simulink library "wt_blockset_beta"  (Simulink 5.0)
values from neighbouring files (symbols this model uses):
  a = -Le\Re    [matrix_coeff_trafo3limb_abc.m]
  a11 = K2*Rs/Ls    [matrix_coeff_scim_abc.m]    (also in matrix_coeff_spsm_dq.m = -Rs*Ksgm_frd/Ksgm_d; matrix_coeff_trafo_abc.m = K2*Rhv/Lhv; matrix_coeff_wrim_abc.m)
  a12 = K3*Rs/Ls    [matrix_coeff_scim_abc.m]    (also in matrix_coeff_spsm_dq.m = Lssq*Ksgm_frd/Ksgm_d; matrix_coeff_trafo_abc.m = K3*Rhv/Lhv; matrix_coeff_wrim_abc.m)
  a13 = 3*Msr*sqrt(3)*K4/4    [matrix_coeff_scim_abc.m]    (also in matrix_coeff_spsm_dq.m = Rf*Lsgm_rd*Lmd/Ksgm_d; matrix_coeff_trafo_abc.m = K4*Rhv; matrix_coeff_wrim_abc.m)
  a14 = K4*Rr    [matrix_coeff_scim_abc.m]    (also in matrix_coeff_spsm_dq.m = Rrd*Lsgm_f*Lmd/Ksgm_d; matrix_coeff_trafo_abc.m = K2/Lhv; matrix_coeff_wrim_abc.m)
  a15 = Msr*(K2-K3)/Ls    [matrix_coeff_scim_abc.m]    (also in matrix_coeff_spsm_dq.m = Lmq*Ksgm_frd/Ksgm_d; matrix_coeff_trafo_abc.m = K3/Lhv; matrix_coeff_wrim_abc.m)
  a16 = K2/Ls    [matrix_coeff_scim_abc.m]    (also in matrix_coeff_spsm_dq.m = Ksgm_frd/Ksgm_d; matrix_coeff_trafo_abc.m = K4; matrix_coeff_wrim_abc.m)
  a17 = K3/Ls    [matrix_coeff_scim_abc.m]    (also in matrix_coeff_spsm_dq.m = -Lsgm_rd*Lmd/Ksgm_d; matrix_coeff_wrim_abc.m)
  a21 = -Lssd*Lsrq/Ksgm_q    [matrix_coeff_spsm_dq.m]
  a22 = -Rs*Lsrq/Ksgm_q    [matrix_coeff_spsm_dq.m]
  a23 = -Lsrq*Lmd/Ksgm_q    [matrix_coeff_spsm_dq.m]
  a24 = -Lsrq*Lmd/Ksgm_q    [matrix_coeff_spsm_dq.m]
  a25 = Rrq*Lmq/Ksgm_q    [matrix_coeff_spsm_dq.m]
  a26 = Lsrq/Ksgm_q    [matrix_coeff_spsm_dq.m]
  a31 = K4*Rs    [matrix_coeff_scim_abc.m]    (also in matrix_coeff_spsm_dq.m = +Rs*Lsgm_rd*Lmd/Ksgm_d; matrix_coeff_trafo_abc.m = K4*Rlv; matrix_coeff_wrim_abc.m)
  a32 = Msr*(K2-K3)/Lr    [matrix_coeff_scim_abc.m]    (also in matrix_coeff_spsm_dq.m = -Lssq*Lsgm_rd*Lmd/Ksgm_d; matrix_coeff_trafo_abc.m = K2*Rlv/Llv; matrix_coeff_wrim_abc.m)
  a33 = K2*Rr/Lr    [matrix_coeff_scim_abc.m]    (also in matrix_coeff_spsm_dq.m = -Rf*Ksgm_srd/Ksgm_d; matrix_coeff_trafo_abc.m = K3*Rlv/Llv; matrix_coeff_wrim_abc.m)
  a34 = K3*Rr/Lr    [matrix_coeff_scim_abc.m]    (also in matrix_coeff_spsm_dq.m = Rrd*Lsgm_s*Lmd/Ksgm_d; matrix_coeff_trafo_abc.m = K4; matrix_coeff_wrim_abc.m)
  a35 = 3*Msr*sqrt(3)*K4/4    [matrix_coeff_scim_abc.m]    (also in matrix_coeff_spsm_dq.m = -Lsgm_rd*Lmd*Lmq/Ksgm_d; matrix_coeff_trafo_abc.m = K2/Llv; matrix_coeff_wrim_abc.m)
  a36 = K4    [matrix_coeff_scim_abc.m]    (also in matrix_coeff_spsm_dq.m = -Lsgm_rd*Lmd/Ksgm_d; matrix_coeff_trafo_abc.m = K3/Llv; matrix_coeff_wrim_abc.m)
  a37 = Ksgm_srd/Ksgm_d    [matrix_coeff_spsm_dq.m]    (also in matrix_coeff_wrim_abc.m = K2/Lr)
  a41 = Rs*Lsgm_f*Lmd/Ksgm_d    [matrix_coeff_spsm_dq.m]
  a42 = -Lsgm_f*Lssq*Lmd/Ksgm_d    [matrix_coeff_spsm_dq.m]
  a43 = Rf*Lsgm_s*Lmd/Ksgm_d    [matrix_coeff_spsm_dq.m]
  a44 = -Rrd*Ksgm_sf/Ksgm_d    [matrix_coeff_spsm_dq.m]
  a45 = -Lsgm_f*Lmd*Lmq/Ksgm_d    [matrix_coeff_spsm_dq.m]
  a46 = -Lsgm_f*Lmd/Ksgm_d    [matrix_coeff_spsm_dq.m]
  a47 = -Lsgm_s*Lmd/Ksgm_d    [matrix_coeff_spsm_dq.m]
  a51 = Lssd*Lmq/Ksgm_q    [matrix_coeff_spsm_dq.m]
  a52 = Rs*Lmq/Ksgm_q    [matrix_coeff_spsm_dq.m]
  a53 = Lmd*Lmq/Ksgm_q    [matrix_coeff_spsm_dq.m]
  a54 = Lmd*Lmq/Ksgm_q    [matrix_coeff_spsm_dq.m]
  a55 = -Rrq*Lssq/Ksgm_q    [matrix_coeff_spsm_dq.m]
  a56 = -Lmq/Ksgm_q    [matrix_coeff_spsm_dq.m]
  alpha_T = Ubase_hv/Ubase_lv    [matrix_coeff_trafo3limb_abc.m]
  b = inv(Le)    [matrix_coeff_trafo3limb_abc.m]
  Ctorque = cq(2:5:102,2:5:182)    [cq_table.m]
  Lmd = mag_ind(1)    [matrix_coeff_spsm_dq.m]
  Lmq = mag_ind(2)    [matrix_coeff_spsm_dq.m]
  Lss = Lsgms+Lm    [init_dbe_dq_scim.m]
  omg_base = 2*pi*rated_fp(1)    [init_dbe_dq_scim.m]    (also in init_dbe_rms_scim.m)
  p = rated_fp(2)    [init_dbe_dq_scim.m]    (also in init_dbe_rms_scim.m)
  Rs = stator(1)    [init_dbe_dq_scim.m]    (also in init_dbe_rms_scim.m; matrix_coeff_scim_abc.m; matrix_coeff_spsm_dq.m = stator_winding(1); matrix_coeff_wrim_abc.m)
  Xs = omg_base*Lss    [init_dbe_dq_scim.m]    (also in init_dbe_rms_scim.m = Xsgm_s+Xm)
undefined symbols (not defined in the file or in its folder): get, j, Kmode, ModeOp, Type, u0
libraries: simulink_extras x12, simulink x4, dspinverses x1, dspmtrx3 x1, dspsigattribs x1, dspspect3 x1
(part 1 of 4)
settings Model: Creator=Florin iov  LastModifiedBy=fi  ModifiedComment=fi -- Tue Jun 01 12:17:17 2004 -- Version beta 1

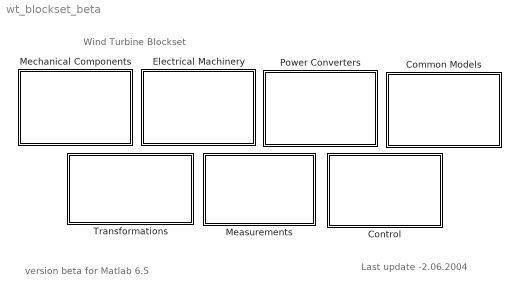
== system wt_blockset_beta ==
  note: Wind Turbine Blockset
  note: Last update -2.06.2004
  note: version beta for Matlab 6.5
  Common Models : Subsystem
      mask Display: disp('Common\nModels')
  Control : Subsystem
      mask Display: disp('Control')
  Electrical Machinery : Subsystem
      mask Display: disp('Electrical\nMachinery')
  Measurements : Subsystem
      mask Display: disp('Measurements')
  Mechanical Components : Subsystem
      mask Display: disp('Mechanical\nComponents')
  Power Converters : Subsystem
      mask Display: disp('Power\nConverters')
  Transformations : Subsystem
      mask Display: disp('Transformations')

== system wt_blockset_beta/Common Models ==
  note: Sources
  note: Cables & Distribution Lines
  note: others
  note: Transformers
  3-phase 3 limb  C S-Function : Subsystem  mask(ABC/abc Dynamic Model of 3-phase 3 limb transformer){power=[2e6 3000], voltage=[30000 690/sqrt(3)], frequency=50, hv_winding=[4.5 51], lv_winding=[3 51], core_ratio=0.33}
      mask prompts: power "Rated power, No-load losses [Sr (VA), Po (W)]"; voltage "Rated phase voltages [U1r (V), U2r (V)]]"; frequency "Rated frequency [Hz]"; hv_winding "High-voltage windings [Rhv  X_hv] [ohms]"; lv_winding "Low-voltage windings [Rlv X_lv] [ohms]"; core_ratio "Core ratio (l/L)"
      mask help:
      | Implements a dynamic model of a 3-phase 2-windings transformer in natural frame (ABC/abc). Core geometry is taken into account.
      | Connection Type Dyn1.
      mask init:
      | matrix_coeff_trafo3limb_abc
      | init_cond = [0 0 0 0 0 0];
      mask Display: disp('3phase 3 limb\n Transformer')
  3-phase 3 limb  Transformer : Subsystem  mask(ABC/abc Dynamic Model of 3-phase 3 limb transformer){power=[2e6 3000], voltage=[30000 690/sqrt(3)], frequency=50, hv_winding=[4.5 51], lv_winding=[3 51], core_ratio=0.33}
      mask prompts: power "Rated power, No-load losses [Sr (VA), Po (W)]"; voltage "Rated phase voltages [U1r (V), U2r (V)]]"; frequency "Rated frequency [Hz]"; hv_winding "High-voltage windings [Rhv  X_hv] [ohms]"; lv_winding "Low-voltage windings [Rlv X_lv] [ohms]"; core_ratio "Core ratio (l/L)"
      mask help:
      | Implements a dynamic model of a 3-phase 2-windings transformer in natural frame (ABC/abc). Core geometry is taken into account.
      | Connection Type Dyn1.
      mask init:
      | matrix_coeff_trafo3limb_abc
      mask Display: disp('3phase 3 limb\n Transformer')
  3-phase line : Subsystem  mask(3-phase distribution line){d=3.3, R=0.115, L=0.19/314, C=0.52e-6}
      mask prompts: d "Line length [km]"; R "Line resistance [ohms/km]"; L "Line inductance [H/km]"; C "Line capacitance [F/km]"
      mask init:
      | Zc=sqrt(L/C);
      | tdelay=d*sqrt(L*C);
      | atten=exp(-(R/2)*d*sqrt(C/L));
      | buffer_size=20000;
  3-phase source : Subsystem  mask(3 - Phase Voltage Source){Uf=220, fs=50}
      mask prompts: Uf "Phase voltage [V]"; fs "Fundamental frequency [Hz]"
  Capacitor Bank RC : Subsystem  mask(Capacitor Bank RC){R=1, CmF=21.737}
      mask prompts: R "Series rezistor [ohms]"; CmF "Branch Capacitor [mF]"
      mask init:
      | C=CmF*1e-3;
      mask Display: disp('Capacitor\nBank')
  Capacitor Bank RLC : Subsystem  mask(Capacitor Bank RLC){R=0.0001, X=0.00034, CmF=0.0005}
      mask prompts: R "Series rezistor [ohms]"; X "Reactor [ohms]"; CmF "Capacitance [mF]"
      mask init:
      | L=X/(2*pi*50);
      | C=CmF*1e-3;
      mask Display: disp('Capacitor\nBank')
  Circuit breaker : Subsystem  mask{to=1/50, Ro=100, tc=1/50, Rc=100}
      mask prompts: to "Opening time"; Ro "Opening resistance"; tc "Closing time"; Rc "Closing resistance"
  DC-link circuit : Subsystem  mask(DC-link circuit){R=0.001, CuF=21.737}
      mask prompts: R "Series rezistor [ohms]"; CuF "Capacitor [uF]"
      mask init:
      | C=CuF*1e-6;
      mask Display: disp('DC\nLink')
  GRID 1 : Subsystem  mask(3 - Phase Voltage Source){Uf=31500, R=0, X=1.5, fs=50}
      mask prompts: Uf "Phase voltage [V]"; R "Resistance"; X "Reactance"; fs "Fundamental frequency [Hz]"
  GRID 2 : Subsystem  mask(3 - Phase Voltage Source){Uf=31500, R=0.01, X=5, fs=50}
      mask prompts: Uf "Phase voltage [V]"; R "Resistance"; X "Reactance"; fs "Fundamental frequency [Hz]"
  Harmonic Voltage Source : Subsystem  mask(Harmonic Voltage Source){phase_o=178.2, h3=on, h5=on, h7=on, h9=on, h11=on, h13=on}
      mask prompts: phase_o "Initial phase [deg]"; h3 "Insertion of 3rd harmonic"; h5 "Insertion of 5th harmonic"; h7 "Insertion of 7th harmonic"; h9 "Insertion of 9th harmonic"; h11 "Insertion of 11th harmonic"; h13 "Insertion of 13th harmonic"
      mask help: Implements a harmonic voltage source according with Standard EN61000-2-2.
      mask init:
      | gama_0=phase_o*pi/180;
  Voltage source complex : Subsystem  mask(3 - Phase Voltage Source){Uf=960}
      mask prompts: Uf "Phase voltage [V]"

== system wt_blockset_beta/Control ==
  note: Control Blocks
  PI anti wind-up : Subsystem  mask{K=0.09, Ti=0.016, ka=10, maxim=1000, init_cond=2}
      mask prompts: K "Proportional Constant"; Ti "Integrate constant"; maxim "Limits"; init_cond "initial"

== system wt_blockset_beta/Electrical Machinery ==
  note: Electrical Machinery Library
  Simulink Blocks  based Models : Subsystem
      mask Display: disp('Simulink Blocks\n based Models')

== system wt_blockset_beta/Measurements ==
  note: Measurements
  Moving Average Filter : Subsystem  mask(Moving Average Filter){Tav=60, init=10}
      mask prompts: Tav "Averaging time interval [sec]"; init "Initial condition"
      mask help: Implements a Moving average filter in time domain
      mask Display: disp('Moving\nAverage')
  P & Q three phase : Subsystem  mask(Active & Reactive Power ){f=50}
      mask prompts: f "Fundamental frequency (Hz):"
      mask Display: disp('P&Q\n 3-phase')
  Phase Locked Loop : Subsystem  mask(Phase Locked Loop){fs=50, Kp=180.03, Ti=0.00786}
      mask prompts: fs "Fundamental frequency (Hz):"; Kp "Proportional coefficient"; Ti "Integration time constant [sec]"
      mask help: Implements a Phase Locked Loop for grid angle detection
      mask Display: disp('PLL')
  power spectra : Subsystem  mask(power spectra){t_sample=0.05}
      mask prompts: t_sample "Sample period"

== system wt_blockset_beta/Mechanical Components ==
  note: Wind Models
  note: Drive Train Models
  note: Rotor Models
  "One-mass model " : Subsystem  mask(Simple Gearbox){Op_Mode=Generator, Jem=90, Jwt=9e6, K=83, init_speed=1.87355}
      mask prompts: Op_Mode "Operation Mode"; Jem "Electric machinery - Moment of inertia [kg m2]"; Jwt "Wind turbine rotor - Moment of inertia [kg*m2]"; K "Gearbox ratio"; init_speed "Initial condition [omg_wt (rad/sec)]"
      mask init:
      | if Op_Mode==1, ModeOp=-1;else ModeOp=1;end
      | J=Jem*K^2+Jwt;
      mask StyleString: popup(Motor|Generator),edit,edit,edit,edit
      mask Display: disp('Drive Train')
  Two-mass model : Subsystem  mask(Gearbox with torsional torque){Jem=90, Jwt=9e6, Kshaft=12e7, Dshaft=3.5e5, Kgear=83, init=[156.5 1.87355]}
      mask prompts: Jem "Electric machine - Moment of inertia:  Jem [ kg*m2]"; Jwt "Wind turbine rotor - Moment of inertia:  Jwt [kg*m2]"; Kshaft "Shaft stiffness:  Kshaft [ Nm/rad]"; Dshaft "Damping coeficient of shaft:  Dshaft [Nm sec/rad]"; Kgear "Gearbox ratio"; init "Initial conditions [omg_em (rad/sec), omg_wt (rad/sec) ]"
      mask help: Implements a gearbox with torsional torque.
      mask Display: disp('Drive Train')
  Two-mass model 'C' S-Function : Subsystem  mask(Gear box with torsional torques){Jem=90, Jwt=9e6, Kshaft=12e7, Dshaft=3.5e5, Kgear=83, init_cond=[156.5 0 1.87355 0]}
      mask prompts: Jem "Electric machine - Moment of inertia:  Jem [ kg*m2]"; Jwt "Wind turbine rotor - Moment of inertia:  Jwt [kg*m2]"; Kshaft "Shaft stiffness:  Kshaft [ Nm/rad]"; Dshaft "Damping coeficient of shaft:  Dshaft [Nm sec/rad]"; Kgear "Gearbox ratio"; init_cond "Initial conditions [omg_em(rad/s) th_em(rad) omg_wtr(rad/s) th_wtr(rad)]"
      mask help:
      | Implemets the dynamic model of a gearbox with torsional torques.
      | Equations are written at the low speed shaft (wind turbine side).
      mask Display: disp('Drive Train')
  Wind Model SB-1 : Subsystem  TreatAsAtomicUnit=on  mask(Wind Model using Simulink Band-limited white noise generator){D_rotor=72, v_mean=10, roughness=600, turb_int=12, T_sample=0.05}
      mask prompts: D_rotor "Rotor diameter [m]"; v_mean "Average wind speed [m/sec]"; roughness "Length scale [m]"; turb_int "Turbulence intensity [%]"; T_sample "Sample time [sec]"
      mask help:
      | Implements a rotor wind model developped by RISOE National Laboratory based on Kaimal spectra. The model takes into account the rotational turbulences and the tower shadow.
      | This model uses the built-in band-limited white noise generator from Simulink
      mask init:
      | r = D_rotor/2;
      | sigma = v_mean*turb_int/100;
      | var = sigma^2;
      | c = roughness/(2*pi*v_mean);
      | d = r/v_mean;
      | trans=sigma*sqrt(roughness/v_mean);
      mask Display: disp('Wind\nModel\n(SB-1)')
  Wind Model SB-2 : Subsystem  TreatAsAtomicUnit=on  mask(Wind Model using Simulink Band-limited white noise generator){D_rotor=72, L=600, turb_int=12, T_sample=0.05}
      mask prompts: D_rotor "Rotor diameter [m]"; L "Length scale [m]"; turb_int "Turbulence intensity [%]"; T_sample "Sample time [sec]"
      mask help:
      | Implements a rotor wind model developped by RISOE National Laboratory based on Kaimal spectra. The model takes into account the rotational turbulences and the tower shadow.
      | This model uses the built-in band-limited white noise generator from Simulink
      mask init:
      | r = D_rotor/2;
      mask Display: disp('Wind\nModel\n(SB-2)')
  Wind Turbine Rotor : Subsystem  mask(Aerodynamic model for wind turbine){R=40, ro_air=1.25, cut_in=3, cut_out=25, Tact=0}
      mask prompts: R "Blade radius [m]"; ro_air "Air density [kg m3]"; cut_in "Cut in speed [m/sec]"; cut_out "Cut out speed [m/sec]"; Tact "Time constant for pitch actuator [sec]"
      mask init:
      | cq_table
      mask Display: plot(20,0,120,200,[45,35,35,45,75,75,45],[85,92,108,115,115,85,85],[55,50,70,65],[115,180,190,115],[55,50,70,65],[85,10,20,85],[75,85],[102,102],[75,85],[98,98],[105,85,85,105],[80,85,115,120])

== system wt_blockset_beta/Power Converters ==
  note: Power Converters Models
  note: Modulation Strategies
  3-phase Diode Bridge Rectifier : Subsystem
      mask Type: 3 phase Diode Bridge Rectifier
      mask Description: Implements a model for 3 phase Diode Bridge Rectifier.
      mask Display: disp('')
  Average PWM Strategy : Subsystem  mask(Average sinusoidal PWM Strategy with Simulink Blocks){third=on}
      mask prompts: third "Insertion of third harmonic"
      mask help: Implements an average model of a sinusoidal PWM strategy using Simulink Blocks.
      mask Display: disp('Average\nPWM')
  Average SVM Strategy : Subsystem
      mask Type: Average SVM Strategy with Simulink Blocks
      mask Description: Implements an average model of a SV-PWM strategy using Simulink Blocks.
      mask Display: disp('Average\nSVM')
  Switching PWM Strategy : Subsystem  mask(Switching sinusoidal PWM with Simulink Blocks){carrier=1000, dead_time=3.2e-6, min_pw=5e-6, dp=on, third=on}
      mask prompts: carrier "Carrier frequency [Hz]"; dead_time "Dead time [sec]"; min_pw "Minimum pulse width [sec]"; dp "Pulse dropping"; third "Insertion of third harmonic"
      mask help: Implements a switching model of a sinusoidal PWM strategy using Simulink Blocks.
      mask init:
      | mpw=0.5*min_pw;
      mask Display: disp('Switching\nPWM')
  Switching SVM Strategy : Subsystem  mask(Switching SVM Strategy with Simulink Blocks){fsw=4000, dead_time=3.2e-6, min_pw=5e-6, dp=off}
      mask prompts: fsw "Switching frequency"; dead_time "Dead time [sec]"; min_pw "Minimum pulse width [sec]"; dp "Pulse dropping"
      mask help: Implements a switching model of a SV-PWM strategy using Simulink Blocks.
      mask init:
      | Tsw=1/fsw;
      | mpw=0.5*min_pw;
      mask Display: disp('Switching\nSVM')
  Voltage Source Converter : Subsystem
      mask Type: Voltage Source Converter - star connected loads
      mask Description:
      | Implements a Voltage Source Converter (Rectifier or Inverter)
      | using switching functions.
      | - input S_ABC is          discret (0,1) => switching model.
      | - input S_ABC is continuous (0...1) =>   average model.
      mask Display: disp('VSC')

== system wt_blockset_beta/Transformations ==
  note: Transformations
  ABC->Mag&Phase : Subsystem
      mask Type: RMS&phase calculator
      mask Description: Calculate the RMS value and phase angle for a 3 phase input.
      mask Display: disp('')
  "DQ -> Complex" : Subsystem
      mask Type: DQ -> Complex
      mask Description: Transformation of dq variables into complex form
  "abc -> dq0" : Subsystem
      mask Description: Implements  ABC -> DQ  transformation
  "dq0 -> abc" : Subsystem
      mask Type: DQ -> ABC
      mask Description: Implements DQ -> ABC transformation
      mask Display: disp(' ')
  "phase -> line currents" : Subsystem
      mask Type: Transformation phase to line currents
      mask Description: Transformation of phase currents into line currents
      mask Display: disp('')
  phase->line voltages : Subsystem
      mask Type: Transformation phase to line voltages
      mask Description: Transformation of phase currents into line voltages
      mask Display: disp('')

== system wt_blockset_beta/Common Models/3-phase 3 limb  C S-Function ==
  v_UVW : Inport
  i_uvw : Inport  Port=2
  Mux : Mux  Inputs=2
  Ropen : Gain  Orientation=down  Gain=1000000  SaturateOnIntegerOverflow=on
  Ropen1 : Gain  Gain=-sqrt(3)  SaturateOnIntegerOverflow=on
  S-Function : S-Function  FunctionName=trafo3limb_abc  Parameters=a b init_cond
  Selector iABC : Selector  Elements=[1 2 3]  InputPortWidth=6
  Selector iabc : Selector  Elements=[4 5 6]  InputPortWidth=6
  Sum : Sum  Inputs=|+-  SaturateOnIntegerOverflow=on  InputSameDT=on
  phase->line2 : Subsystem
  turns ratio : Gain  Gain=-alpha_T  SaturateOnIntegerOverflow=on
  turns ratio1 : Gain  Gain=alpha_T  SaturateOnIntegerOverflow=on
  i_UVW : Outport
  v_uvw : Outport  Port=2
  wires:
  i_uvw/1 -> Sum/2
  turns ratio1/1 -> Sum/1
  Ropen1/1 -> v_uvw/1
  Ropen/1 -> turns ratio/1, Ropen1/1
  Sum/1 -> Ropen/1
  S-Function/1 -> Selector iabc/1, Selector iABC/1
  Mux/1 -> S-Function/1
  turns ratio/1 -> Mux/2
  v_UVW/1 -> Mux/1
  phase->line2/1(out) -> i_UVW/1
  Selector iABC/1 -> phase->line2/1(in)
  Selector iabc/1 -> turns ratio1/1

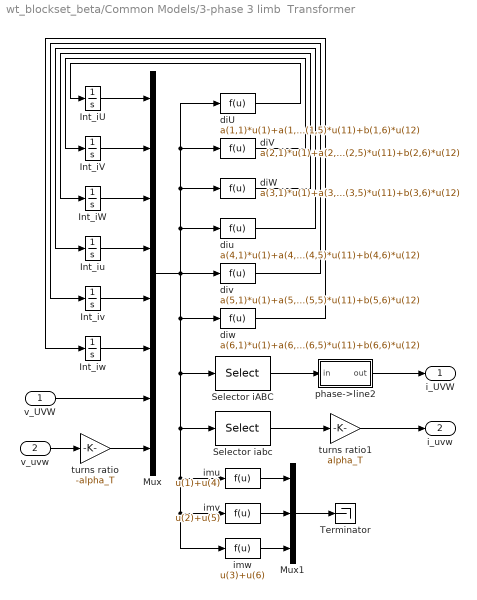
== system wt_blockset_beta/Common Models/3-phase 3 limb  Transformer ==
  v_UVW : Inport
  v_uvw : Inport  Port=2
  Int_iU : Integrator
  Int_iV : Integrator
  Int_iW : Integrator
  Int_iu : Integrator
  Int_iv : Integrator
  Int_iw : Integrator
  Mux : Mux  Inputs=[1 1 1 1 1 1 3 3]
  Mux1 : Mux  Inputs=3
  Selector iABC : Selector  Elements=[1 2 3]  InputPortWidth=12
  Selector iabc : Selector  Elements=[4 5 6]  InputPortWidth=12
  Terminator : Terminator
  diU : Fcn  Expr=a(1,1)*u(1)+a(1,2)*u(2)+a(1,3)*u(3)+a(1,4)*u(4)+a(1,5)*u(5)+a(1,6)*u(6)+b(1,1)*u(7)+b(1,2)*u(8)+b(1,3)*u(9)+b(1,4)*u(10)+b(1,5)*u(11)+b(1,6)*u(12)
  diV : Fcn  Expr=a(2,1)*u(1)+a(2,2)*u(2)+a(2,3)*u(3)+a(2,4)*u(4)+a(2,5)*u(5)+a(2,6)*u(6)+b(2,1)*u(7)+b(2,2)*u(8)+b(2,3)*u(9)+b(2,4)*u(10)+b(2,5)*u(11)+b(2,6)*u(12)
  diW : Fcn  Expr=a(3,1)*u(1)+a(3,2)*u(2)+a(3,3)*u(3)+a(3,4)*u(4)+a(3,5)*u(5)+a(3,6)*u(6)+b(3,1)*u(7)+b(3,2)*u(8)+b(3,3)*u(9)+b(3,4)*u(10)+b(3,5)*u(11)+b(3,6)*u(12)
  diu : Fcn  Expr=a(4,1)*u(1)+a(4,2)*u(2)+a(4,3)*u(3)+a(4,4)*u(4)+a(4,5)*u(5)+a(4,6)*u(6)+b(4,1)*u(7)+b(4,2)*u(8)+b(4,3)*u(9)+b(4,4)*u(10)+b(4,5)*u(11)+b(4,6)*u(12)
  div : Fcn  Expr=a(5,1)*u(1)+a(5,2)*u(2)+a(5,3)*u(3)+a(5,4)*u(4)+a(5,5)*u(5)+a(5,6)*u(6)+b(5,1)*u(7)+b(5,2)*u(8)+b(5,3)*u(9)+b(5,4)*u(10)+b(5,5)*u(11)+b(5,6)*u(12)
  diw : Fcn  Expr=a(6,1)*u(1)+a(6,2)*u(2)+a(6,3)*u(3)+a(6,4)*u(4)+a(6,5)*u(5)+a(6,6)*u(6)+b(6,1)*u(7)+b(6,2)*u(8)+b(6,3)*u(9)+b(6,4)*u(10)+b(6,5)*u(11)+b(6,6)*u(12)
  imu : Fcn  Expr=u(1)+u(4)
  imv : Fcn  Expr=u(2)+u(5)
  imw : Fcn  Expr=u(3)+u(6)
  phase->line2 : Subsystem
  turns ratio : Gain  Gain=-alpha_T  SaturateOnIntegerOverflow=on
  turns ratio1 : Gain  Gain=alpha_T  SaturateOnIntegerOverflow=on
  i_UVW : Outport
  i_uvw : Outport  Port=2
  wires:
  turns ratio/1 -> Mux/8
  Selector iabc/1 -> turns ratio1/1
  Selector iABC/1 -> phase->line2/1(in)
  v_uvw/1 -> turns ratio/1
  v_UVW/1 -> Mux/7
  diw/1 -> Int_iw/1
  div/1 -> Int_iv/1
  diu/1 -> Int_iu/1
  diW/1 -> Int_iW/1
  diV/1 -> Int_iV/1
  diU/1 -> Int_iU/1
  Int_iw/1 -> Mux/6
  Int_iv/1 -> Mux/5
  Int_iu/1 -> Mux/4
  Int_iW/1 -> Mux/3
  Int_iV/1 -> Mux/2
  Int_iU/1 -> Mux/1
  Mux/1 -> Selector iABC/1, Selector iabc/1, imu/1, imv/1, imw/1, diw/1, div/1, diU/1, diV/1, diW/1, diu/1
  turns ratio1/1 -> i_uvw/1
  phase->line2/1(out) -> i_UVW/1
  imu/1 -> Mux1/1
  imv/1 -> Mux1/2
  imw/1 -> Mux1/3
  Mux1/1 -> Terminator/1

== system wt_blockset_beta/Common Models/3-phase line ==
  note: VfR
  note: VbR
  note: VfS
  note: VbS
  iS_abc : Inport
  iR_abc : Inport  Orientation=left  Port=2
  1 : Gain  Gain=atten  SaturateOnIntegerOverflow=on
  2 : Gain  Orientation=left  Gain=atten  SaturateOnIntegerOverflow=on
  Gain1 : Gain  Orientation=left  Gain=2  SaturateOnIntegerOverflow=on
  Gain6 : Gain  Gain=2  SaturateOnIntegerOverflow=on
  R_to_S delay : TransportDelay  Orientation=left  DelayTime=tdelay  BufferSize=buffer_size
  S_to_R delay : TransportDelay  DelayTime=tdelay  BufferSize=buffer_size
  Sum1 : Sum  Orientation=up  SaturateOnIntegerOverflow=on  InputSameDT=on
  Sum2 : Sum  Inputs=+-  SaturateOnIntegerOverflow=on  InputSameDT=on
  Sum4 : Sum  Orientation=down  Inputs=+-  SaturateOnIntegerOverflow=on  InputSameDT=on
  Sum5 : Sum  Orientation=left  Inputs=-+  SaturateOnIntegerOverflow=on  InputSameDT=on
  Zc1 : Gain  Orientation=up  Gain=Zc  SaturateOnIntegerOverflow=on
  Zc2 : Gain  Orientation=down  Gain=Zc  SaturateOnIntegerOverflow=on
  VS_abc : Outport  Orientation=left  InitialOutput=0
  "VR_abc " : Outport  Port=2  InitialOutput=0
  wires:
  1/1 -> Sum5/1, Gain6/1
  Sum1/1 -> Sum2/1, VS_abc/1
  iR_abc/1 -> Zc2/1
  iS_abc/1 -> Zc1/1
  Sum4/1 -> "VR_abc "/1, Sum5/2
  Sum5/1 -> R_to_S delay/1
  Zc2/1 -> Sum4/2
  Sum2/1 -> S_to_R delay/1
  Zc1/1 -> Sum1/1
  Gain6/1 -> Sum4/1
  Gain1/1 -> Sum1/2
  S_to_R delay/1 -> 1/1
  R_to_S delay/1 -> 2/1
  2/1 -> Gain1/1, Sum2/2

== system wt_blockset_beta/Common Models/3-phase source ==
  Mux3 : Mux  Inputs=3
  ua : Sin  Amplitude=sqrt(2)*Uf  Frequency=2*pi*fs  SampleTime=0
  ub : Sin  Amplitude=sqrt(2)*Uf  Frequency=2*pi*fs  Phase=-2*pi/3  SampleTime=0
  uc : Sin  Amplitude=sqrt(2)*Uf  Frequency=2*pi*fs  Phase=2*pi/3  SampleTime=0
  uRST : Outport  InitialOutput=0
  wires:
  uc/1 -> Mux3/3
  ub/1 -> Mux3/2
  Mux3/1 -> uRST/1
  ua/1 -> Mux3/1

== system wt_blockset_beta/Common Models/Capacitor Bank RC ==
  V_RST : Inport
  k : Inport  Port=2
  Branch A : TransferFcn  Numerator=[C 0]  Denominator=[R*C 1]
  Branch B : TransferFcn  Numerator=[C 0]  Denominator=[R*C 1]
  Branch C : TransferFcn  Numerator=[C 0]  Denominator=[R*C 1]
  Demux : Demux  Outputs=3
  Mux : Mux  Inputs=3
  Product : Product  SaturateOnIntegerOverflow=on  InputSameDT=on
  I_RST : Outport
  wires:
  k/1 -> Product/2
  Product/1 -> I_RST/1
  V_RST/1 -> Demux/1
  Mux/1 -> Product/1
  Branch C/1 -> Mux/3
  Branch B/1 -> Mux/2
  Branch A/1 -> Mux/1
  Demux/3 -> Branch C/1
  Demux/2 -> Branch B/1
  Demux/1 -> Branch A/1

== system wt_blockset_beta/Common Models/Capacitor Bank RLC ==
  v_RST : Inport
  k : Inport  Port=2
  Demux : Demux  Outputs=3
  Mux : Mux  Inputs=3
  Product : Product  SaturateOnIntegerOverflow=on  InputSameDT=on
  Transfer Fcn : TransferFcn  Numerator=[C 0]  Denominator=[L*C R*C 1]
  Transfer Fcn1 : TransferFcn  Numerator=[C 0]  Denominator=[L*C R*C 1]
  Transfer Fcn2 : TransferFcn  Numerator=[C 0]  Denominator=[L*C R*C 1]
  I_RST : Outport
  wires:
  v_RST/1 -> Demux/1
  Transfer Fcn2/1 -> Mux/3
  Transfer Fcn1/1 -> Mux/2
  Transfer Fcn/1 -> Mux/1
  Demux/1 -> Transfer Fcn/1
  Demux/2 -> Transfer Fcn1/1
  Demux/3 -> Transfer Fcn2/1
  k/1 -> Product/2
  Product/1 -> I_RST/1
  Mux/1 -> Product/1

== system wt_blockset_beta/Common Models/Circuit breaker ==
  Vin_ABC : Inport  Orientation=left
  Is_ABC : Inport  Orientation=left  Port=2
  CB : Inport  Orientation=left  Port=3
  Circuit breaker1 : Subsystem  Orientation=left
  Circuit breaker2 : Subsystem  Orientation=left
  Circuit breaker3 : Subsystem  Orientation=left
  Demux : Demux  Orientation=left  Outputs=3
  Demux1 : Demux  Orientation=left  Outputs=3
  Mux : Mux  Orientation=left  Inputs=3
  Vb_ABC : Outport  Orientation=left
  wires:
  Mux/1 -> Vb_ABC/1
  Circuit breaker3/1(vc) -> Mux/3
  Circuit breaker1/1(va) -> Mux/1
  Circuit breaker2/1(vb) -> Mux/2
  CB/1 -> Circuit breaker3/3(on/off), Circuit breaker2/3(on/off), Circuit breaker1/3(on/off)
  Demux1/3 -> Circuit breaker3/2(iT)
  Demux1/2 -> Circuit breaker2/2(iR)
  Demux1/1 -> Circuit breaker1/2(iS)
  Is_ABC/1 -> Demux1/1
  Demux/3 -> Circuit breaker3/1(Vin)
  Demux/1 -> Circuit breaker1/1(Vin)
  Vin_ABC/1 -> Demux/1
  Demux/2 -> Circuit breaker2/1(Vin)

== system wt_blockset_beta/Common Models/DC-link circuit ==
  idc_inv : Inport
  idc_red : Inport  Port=2
  DC capacitor : TransferFcn  Numerator=[R C]  Denominator=[1 0]
  Sum : Sum  Inputs=|+-  SaturateOnIntegerOverflow=on  InputSameDT=on
  vdc : Outport
  wires:
  DC capacitor/1 -> vdc/1
  Sum/1 -> DC capacitor/1
  idc_inv/1 -> Sum/2
  idc_red/1 -> Sum/1

== system wt_blockset_beta/Common Models/GRID 1 ==
  uRST : Inport
  Gain : Gain  Gain=X/(2*pi*fs)  SaturateOnIntegerOverflow=on
  Gain1 : Gain  Orientation=left  Gain=R  SaturateOnIntegerOverflow=on
  Integrator : Integrator
  Mux3 : Mux  Inputs=3
  Sum : Sum  Inputs=-+-  SaturateOnIntegerOverflow=on  InputSameDT=on
  ua : Sin  Amplitude=sqrt(2)*Uf  Frequency=2*pi*fs  SampleTime=0
  ub : Sin  Amplitude=sqrt(2)*Uf  Frequency=2*pi*fs  Phase=-2*pi/3  SampleTime=0
  uc : Sin  Amplitude=sqrt(2)*Uf  Frequency=2*pi*fs  Phase=2*pi/3  SampleTime=0
  iRST : Outport  InitialOutput=0
  wires:
  ua/1 -> Mux3/1
  ub/1 -> Mux3/2
  uc/1 -> Mux3/3
  Sum/1 -> Gain/1
  Integrator/1 -> iRST/1, Gain1/1
  Mux3/1 -> Sum/2
  uRST/1 -> Sum/1
  Gain/1 -> Integrator/1
  Gain1/1 -> Sum/3

== system wt_blockset_beta/Common Models/GRID 2 ==
  i_RST : Inport
  Derivative : Derivative
  Gain : Gain  Gain=X/(2*pi*fs)  SaturateOnIntegerOverflow=on
  Gain1 : Gain  Gain=R  SaturateOnIntegerOverflow=on
  Mux3 : Mux  Inputs=3
  Sum : Sum  SaturateOnIntegerOverflow=on  InputSameDT=on
  Sum1 : Sum  SaturateOnIntegerOverflow=on  InputSameDT=on
  ua : Sin  Amplitude=sqrt(2)*Uf  Frequency=2*pi*fs  SampleTime=0
  ub : Sin  Amplitude=sqrt(2)*Uf  Frequency=2*pi*fs  Phase=-2*pi/3  SampleTime=0
  uc : Sin  Amplitude=sqrt(2)*Uf  Frequency=2*pi*fs  Phase=2*pi/3  SampleTime=0
  u_RST : Outport  InitialOutput=0
  wires:
  Sum1/1 -> u_RST/1
  Mux3/1 -> Sum1/1
  Sum/1 -> Sum1/2
  Gain1/1 -> Sum/1
  Derivative/1 -> Sum/2
  Gain/1 -> Derivative/1
  i_RST/1 -> Gain/1, Gain1/1
  ua/1 -> Mux3/1
  ub/1 -> Mux3/2
  uc/1 -> Mux3/3

== system wt_blockset_beta/Common Models/Harmonic Voltage Source ==
  ampl : Inport
  freq : Inport  Port=2
  phase : Inport  Port=3
  Gain : Gain  Gain=2*pi  SaturateOnIntegerOverflow=on
  Integrator : Integrator
  Mux1 : Mux  Inputs=3
  Mux2 : Mux  Inputs=2
  Phase A : Subsystem
  Phase B : Subsystem
  Phase C : Subsystem
  Sum1 : Sum  Inputs=|++  SaturateOnIntegerOverflow=on
  v_RSTh : Outport
  gama : Outport  Port=2
  wires:
  freq/1 -> Gain/1
  ampl/1 -> Mux2/1
  Gain/1 -> Integrator/1
  Mux1/1 -> v_RSTh/1
  Phase A/1(v_harm) -> Mux1/1
  Phase B/1(v_harm) -> Mux1/2
  Phase C/1(v_harm) -> Mux1/3
  Mux2/1 -> Phase B/1(Input), Phase A/1(Input), Phase C/1(Input)
  Integrator/1 -> Sum1/1
  Sum1/1 -> Mux2/2
  phase/1 -> Sum1/2
  [gama] -> gama/1

== system wt_blockset_beta/Common Models/Voltage source complex ==
  Constant : Constant  Value=sqrt(2)*Uf
  Constant1 : Constant  Value=pi/2
  Magnitude-Angle to Complex : MagnitudeAngleToComplex
  V_c : Outport  InitialOutput=0
  wires:
  Constant1/1 -> Magnitude-Angle to Complex/2
  Constant/1 -> Magnitude-Angle to Complex/1
  Magnitude-Angle to Complex/1 -> V_c/1

== system wt_blockset_beta/Control/PI anti wind-up ==
  ref : Inport
  meas : Inport  Port=2
  1/T : Gain  Gain=1/Ti  SaturateOnIntegerOverflow=on
  Integrator : Integrator  InitialCondition=init_cond
  P1 : Gain  Gain=K  SaturateOnIntegerOverflow=on
  P2 : Gain  Orientation=left  Gain=ka  SaturateOnIntegerOverflow=on
  Saturation : Saturate  UpperLimit=maxim  LowerLimit=-maxim
  Sum1 : Sum  Inputs=|+-  SaturateOnIntegerOverflow=on  InputSameDT=on
  Sum2 : Sum  Inputs=++|  SaturateOnIntegerOverflow=on  InputSameDT=on
  Sum3 : Sum  Inputs=|+-  SaturateOnIntegerOverflow=on  InputSameDT=on
  Sum4 : Sum  Orientation=left  Inputs=+-|  SaturateOnIntegerOverflow=on  InputSameDT=on
  out : Outport  InitialOutput=0
  wires:
  Sum1/1 -> 1/T/1
  Integrator/1 -> Sum2/2
  1/T/1 -> Integrator/1
  Sum3/1 -> P1/1
  ref/1 -> Sum3/1
  P1/1 -> Sum1/1, Sum2/1
  meas/1 -> Sum3/2
  P2/1 -> Sum1/2
  Sum2/1 -> Sum4/1, Saturation/1
  Sum4/1 -> P2/1
  Saturation/1 -> out/1, Sum4/2

== system wt_blockset_beta/Electrical Machinery/Simulink Blocks  based Models ==
  note: Electric Machines Dynamic Models
  note: RMS Models
  note: Simulink Blocks
      |  based Models
  note: Special Models
  note: DQ Reference frame
  note: Reduced Order Models
  RMS Wound Rotor Induction Machine : Subsystem  mask(Complex Steady-State Induction Machine){rated_vi=[960 1310], rated_fp=[50 2], standstill=[9 79.5], stator=[0.005 4e-4], rotor=[0.009 3e-4], Lm=16e-3}
      mask prompts: rated_vi "Rated voltage / current per phase [Vph_r (V), Iph_r (A)]"; rated_fp "Base frequency,  Number of pole pairs [fs (Hz), p]"; standstill "Starting current,  Phase angle at standstill [Ist (pu), phi_st (deg)]"; stator "Stator parameters [Rs (ohms), Lsgm_s (H)]"; rotor "Rotor parameters [Rr (ohms), Lsgm_r (H)]"; Lm "Magnetizing inductance [H]"
      mask help:
      | Complex Steady-State Model of Induction Machine.
      | Deep-bar effect taken into account.
      mask init:
      | p=rated_fp(2); omg_synch=2*pi*rated_fp(1);
      | Xm=omg_synch*Lm;
      | Rs=stator(1); Xsgm_s= omg_synch*stator(2); Xs=Xsgm_s+Xm;
      | Rr=rotor(1); Xsgm_r=omg_synch*rotor(2); Xr=Xsgm_r+Xm;
      | sbd=Rr*sqrt((Rs^2+Xs^2)/((Xm^2-Xs*Xr)^2+(Rs*Xr)^2));
      | Rr_sc=(rated_vi(1)*sqrt(1/(1+(tan(standstill(2)*pi/180))^2))/standstill(1)/rated_vi(2)-Rs);
      | kr=Rr_sc/Rr;
      | kx=(tan(standstill(2)*pi/180)*(Rs+Rr_sc)-Xsgm_s)/Xsgm_r;
      mask Display: disp('Steady_State\nModel')
  RMS  Squirrel Cage Induction Machine : Subsystem  mask(Squirrel-Cage Induction Machine){rated_vi=[960 1300], rated_fp=[50 2], standstill=[9 79.5], stator=[0.005 0.13], rotor=[0.009 0.1], Xm=5}
      mask prompts: rated_vi "Rated voltage / current per phase [Vph_r (V), Iph_r (A)]"; rated_fp "Base frequency,  Number of pole pairs [fs (Hz), p]"; standstill "Starting current,  Phase angle at standstill [Ist (pu), phi_st (deg)]"; stator "Stator parameters [Rs Xsgm_s]  [ohms]"; rotor "Rotor parameters [Rr Xsgm_r] [ohms]"; Xm "Magnetizing reactance [ohms]"
      mask help: Steady-State Model of Squirrel-cage Induction Machine
      mask init:
      | init_dbe_rms_scim
      mask Display: disp('Steady_State\nModel')
  Reduced Order Model Induction Machine : Subsystem  mask(Generalized 3rd order model of Asynchronous Generator){stator=[0.0011, 7e-005], rotor=[0.0013, 7.5e-005], magnetization=2.9936e-003, rated_fp=[50 2], init_cond=[0 0]}
      mask prompts: stator "Stator parameters [Rs (ohms), Lsgm_s (H)]"; rotor "Rotor parameters [Rr (ohms), Lsgm_r (H)]"; magnetization "Magnetizing inductance Lm (H)"; rated_fp "Base frequency, Number of pole pairs [fs (Hz), p]"; init_cond "Initial conditions [fi_dr (Wb), fi_qr(Wb)]"
      mask help: Implements a generalized 3rd order model for Asynchronous Generator in synchronous reference frame.
      mask init:
      | Rs=stator(1);Lsgm_s=stator(2);
      | Rr=rotor(1);Lsgm_r=rotor(2);Lm=magnetization;
      | omg_e=2*pi*rated_fp(1);p=rated_fp(2);
      | Lss=Lsgm_s+Lm;Lrr=Lsgm_r+Lm;D=Lss*Lrr-Lm^2;
      | tau_sr=Rs*Lrr/D;tau_rm=Rr*Lm/D;sigma_r=Lm/Lrr;sigma_s=Lm/Lss;
      | alpha=1/(1+(omg_e/tau_sr)^2);
      | M=[Lss 0 Lm 0;0 Lss 0 Lm;Lm 0 Lrr 0;0 Lm 0 Lrr];
      | Q=inv(M);
      mask Display: disp('IM\n3rd Order Model')
  Salient-Pole Synchronous Machine constant parameters : Subsystem  mask{stator_winding=[2.34e-3 3.92e-4], field_winding=[5e-4 6.69246e-4], rotor_winding=[17.36e-3 5.22558e-4 16.75e-3 3.36082e-4], mag_ind=[2.3844e-3 1.1759e-3], p=32}
      mask prompts: stator_winding "Stator winding [Rs Lsgm_s]"; field_winding "Field winding [Rf Lsgm_f]"; rotor_winding "Rotor winding [Rrd Lsgm_rd Rrq Lsgm_rq]"; mag_ind "Magnetizing inductances [Lmd Lmq]"; p "Number of pole pairs"
      mask init:
      | matrix_coeff_spsm_dq
      mask Display: disp('SP_SM')
  Squirrel Cage Induction Machine constant parameters : Subsystem  mask(Squirrel-Cage Induction Machine){Op_Mode=Generator, ConnType=Y, stator=[3.67 9.2e-3], rotor=[2.32 12.29e-3], Lm=0.235, p=2, x0=[0 0 0 0 0]}
      mask prompts: Op_Mode "Operating mode"; ConnType "Connection type"; stator "Stator parameters [Rs (ohm), Lsgm_s(H)]"; rotor "Rotor parameters [Rr (ohm) Lsgm_r (H)]"; Lm "Mutual inductance [H]"; p "Number of pole pairs"; x0 "Initial conditions [ids iqs idr iqr theta]"
      mask help:
      | Implements a dq model in rotor reference frame for squirrel-cage induction machine.
      | Currents as state variable.
      mask init:
      | if ConnType==1,Type=1;else Type=-1;end
      | if Op_Mode==1, Kmode=1;else Kmode=-1;end
      | Rs=stator(1); Lsgms= stator(2); Lss=Lsgms+Lm;
      | Rr=rotor(1); Lsgmr=rotor(2); Lsr=Lsgmr+Lm;
      | sigma=1-(Lm*Lm)/(Lss*Lsr);
      mask Help: web(sc_im)
      mask StyleString: popup(Motor|Generator),popup(Y|D),edit,edit,edit,edit,edit
      mask Display: disp('SC_IM')
  Squirrel Cage  Induction Machine  with Deep Bar Effect : Subsystem  mask(Squirrel-Cage Induction Machine with Deep Bar Effect){Op_Mode=Motor, ConnType=Y, rated_vi=[960 1300], rated_fp=[50 2], standstill=[9 79.5], stator=[0.005 4e-4], rotor=[0.009 3e-4], Lm=16e-3, x0=[0 0 0 0 0]}
      mask prompts: Op_Mode "Operating mode"; ConnType "Connection type"; rated_vi "Rated voltage / current per-phase [Vph_r (V), Iph_r (A)]"; rated_fp "Base frequency,  Number of pole pairs [fs (Hz), p]"; standstill "Starting current,  Phase angle at standstill [Ist (pu), phi_st (deg)]"; stator "Stator [Rs (ohm), Lsgm_s (H)]"; rotor "Rotor [Rr (ohm), Lsgm_r (H)]"; Lm "Magnetizing inductance Lm [H]"; x0 "Initial conditions [ids iqs idr iqr theta]"
      mask help: Implement a DQ Model in rotor reference frame for Squirrel-Cage Induction Machine with Deep bar effect
      mask init:
      | if ConnType==1,Type=1;else Type=-1;end
      | if Op_Mode==1, Kmode=1;else Kmode=-1;end
      | init_dbe_dq_scim
      mask StyleString: popup(Motor|Generator),popup(Y|D),edit,edit,edit,edit,edit,edit,edit
      mask Display: disp('SC_IM')
  Wound Rotor Induction Machine constant parameters : Subsystem  mask(3-phase Wound Rotor Induction Machine){stator=[0.01 95.5e-6], rotor=[0.01 95.5e-6], Lm=0.0955, p=2, x0=[0 0 0 0 0]}
      mask prompts: stator "Stator parameters [Rs (ohm), Lsgm_s (H)]"; rotor "Rotor parameters [Rr (ohm), Lsgm_r (H)]"; Lm "Magnetizing inductance [H]"; p "Number of poles pair"; x0 "Initial conditions [ids iqs idr' iqr' theta]"
      mask init:
      | Rs=stator(1); Lsgm_s=stator(2);
      | Rr=rotor(1); Lsgm_r=rotor(2);
      | Lss=Lsgm_s+Lm;
      | Lsr=Lsgm_r+Lm;
      | sigma=1-(Lm*Lm)/(Lss*Lsr);
      mask Display: disp('WR_IM')
  "Wound Rotor Induction Machine with Deep Bar Effect " : Subsystem  mask(3-phase Wound Rotor Induction Machine){rated_vi=[960 1310], rated_fp=[50 2], standstill=[9 79.5], stator=[0.01 95.5e-6], rotor=[0.01 95.5e-6], Lm=0.0955, x0=[0 0 0 0 0]}
      mask prompts: rated_vi "Rated voltage / current per-phase [Vph_r (V), Iph_r (A)]"; rated_fp "Base frequency,  Number of pole pairs [fs (Hz), p]"; standstill "Starting current,  Phase angle at standstill [Ist (pu), phi_st (deg)]"; stator "Stator [Rs (ohm), Lsgm_s (H)]"; rotor "Rotor [Rr (ohm), Lsgm_r (H)]"; Lm "Magnetizing inductance Lm [H]"; x0 "Initial conditions [ids iqs idr' iqr' theta]"
      mask init:
      | init_dbe_dq_wrim
      mask Display: disp('WR_IM')

== system wt_blockset_beta/Measurements/Moving Average Filter ==
  In : Inport
  Constant : Constant  Value=init
  Gain : Gain  Gain=1/Tav  SaturateOnIntegerOverflow=on
  Integrator : Integrator
  Sum : Sum  Inputs=|+-  SaturateOnIntegerOverflow=on
  Sum1 : Sum  Inputs=|++  SaturateOnIntegerOverflow=on
  Transport Delay : TransportDelay  DelayTime=Tav  InitialInput=init  BufferSize=6144  TransDelayFeedthrough=on
  Out : Outport
  wires:
  In/1 -> Transport Delay/1, Sum/1
  Transport Delay/1 -> Sum/2
  Sum/1 -> Integrator/1
  Integrator/1 -> Gain/1
  Gain/1 -> Sum1/1
  Constant/1 -> Sum1/2
  Sum1/1 -> Out/1

== system wt_blockset_beta/Measurements/P & Q three phase ==
  vabc : Inport
  iabc : Inport  Port=2
  Gain : Gain  Gain=f  SaturateOnIntegerOverflow=on
  Mux : Mux  Inputs=2
  Product1 : Product  SaturateOnIntegerOverflow=on  InputSameDT=on
  Product2 : Product  SaturateOnIntegerOverflow=on  InputSameDT=on
  Sum : Sum  Inputs=+  SaturateOnIntegerOverflow=on
  Sum1 : Sum  Inputs=+-  SaturateOnIntegerOverflow=on  InputSameDT=on
  Sum2 : Sum  Inputs=+  SaturateOnIntegerOverflow=on
  T : TransportDelay  DelayTime=1/f
  T\4 : TransportDelay  DelayTime=1/f/4
  integ : Integrator
  PQ : Outport  InitialOutput=0
  wires:
  Sum2/1 -> Mux/2
  Sum/1 -> Mux/1
  Sum1/1 -> Gain/1
  integ/1 -> T/1, Sum1/1
  T/1 -> Sum1/2
  Mux/1 -> integ/1
  Gain/1 -> PQ/1
  Product1/1 -> Sum2/1
  Product2/1 -> Sum/1
  T\4/1 -> Product1/1
  vabc/1 -> Product2/1, T\4/1
  iabc/1 -> Product2/2, Product1/2

== system wt_blockset_beta/Measurements/Phase Locked Loop ==
  v_RST : Inport
  Integrator : Integrator
  Mux2 : Mux  Inputs=2
  PI anti wind-up2 : Subsystem  mask{K=Kp, Ti=Ti, ka=10, maxim=100, init_cond=0}
      mask prompts: K "Proportional Constant"; Ti "Integrate constant"; maxim "Limits"; init_cond "initial"
  Product : Product  SaturateOnIntegerOverflow=on
  Product1 : Product  SaturateOnIntegerOverflow=on
  Sum : Sum  Inputs=-+  SaturateOnIntegerOverflow=on
  Sum1 : Sum  Inputs=|++  SaturateOnIntegerOverflow=on
  Trigonometric Function : Trigonometry
  Trigonometric Function1 : Trigonometry  Operator=cos
  base freq : Constant  Orientation=up  Value=2*pi*50
  cos(gama) : Fcn  Expr=u(2)/sqrt(u(1)^2+u(2)^2)
  sin(gama) : Fcn  Expr=u(1)/sqrt(u(1)^2+u(2)^2)
  vx : Fcn  Expr=2/3*u(1)-(u(2)+u(3))/3
  vy : Fcn  Expr=-(u(2)-u(3))/sqrt(3)
  theta : Outport  InitialOutput=0
  wires:
  sin(gama)/1 -> Product1/1
  Product/1 -> Sum/1
  Product1/1 -> Sum/2
  Sum/1 -> PI anti wind-up2/1(ref)
  PI anti wind-up2/1(out) -> Sum1/1
  Sum1/1 -> Integrator/1
  Trigonometric Function/1 -> Product/1
  Trigonometric Function1/1 -> Product1/2
  base freq/1 -> Sum1/2
  Integrator/1 -> Trigonometric Function/1, theta/1, Trigonometric Function1/1
  v_RST/1 -> vx/1, vy/1
  cos(gama)/1 -> Product/2
  vy/1 -> Mux2/2
  vx/1 -> Mux2/1
  Mux2/1 -> cos(gama)/1, sin(gama)/1

== system wt_blockset_beta/Measurements/power spectra ==
  Input : Inport
  Spectrum Scope : Subsystem  TreatAsAtomicUnit=on  SimViewingDevice=on  mask(Spectrum Scope){ScopeProperties=on, Domain=Frequency, HorizSpan=1, UseBuffer=on, BufferSize=1024, Overlap=32, inpFftLenInherit=on, FFTlength=1024, numAvg=3, DisplayProperties=off, AxisGrid=on, Memory=off, FrameNumber=on, AxisLegend=off, AxisZoom=off, OpenScopeAtSimStart=on, OpenScopeImmediately=off, FigPos=get(0,'defaultfigureposition'), AxisProperties=off, XUnits=Hertz, XRange=[0...Fs/2], InheritXIncr=off, XIncr=0.05, XLabel=Samples, YUnits=dB, YMin=-80, YMax=80, YLabel=Magnitude, dB, LineProperties=off, LineDisables=, LineStyles=, LineMarkers=, LineColors=[1 0 0]}
      mask prompts: ScopeProperties "-------------------------------- Show scope properties ------------------------------------"; Domain "Input domain:"; HorizSpan "Time display span (number of frames):"; UseBuffer "Buffer input"; BufferSize "Buffer size:"; Overlap "Buffer overlap:"; inpFftLenInherit "Specify FFT length"; FFTlength "FFT length:"; numAvg "Number of spectral averages:"; DisplayProperties "-------------------------------- Show display properties -----------------------------------"; AxisGrid "Show grid"; Memory "Persistence"; FrameNumber "Frame number"; AxisLegend "Channel legend"; AxisZoom "Compact display"; OpenScopeAtSimStart "Open scope at start of simulation"; OpenScopeImmediately "Open scope immediately"; FigPos "Scope position:"; AxisProperties "-------------------------------- Show axis properties ----------------------------------------"; XUnits "Frequency units:"; XRange "Frequency range:"; InheritXIncr "Inherit sample increment from input"; XIncr "Sample time of original time series:"; XLabel "X-axis title:"; YUnits "Amplitude scaling:"; YMin "Minimum Y-limit:"; YMax "Maximum Y-limit:"; YLabel "Y-axis title:"; LineProperties "-------------------------------- Show line properties -----------------------------------------"; LineDisables "Line visibility:"; LineStyles "Line styles:"; LineMarkers "Line markers:"; LineColors "Line colors:"
      mask help: Compute and display the short-time FFT of each input signal. Non-frame based inputs to the block should use the buffering option.
      mask init:
      | [x,y,str] = dspblkbfftscope2('icon');
      | s = dspblkbfftscope2('init');
      settings: DeleteFcn=sdspfscope2([],[],[],'BlockDelete');  NameChangeFcn=sdspfscope2([],[],[],'NameChange');  RTWSystemCode=Function
      settings: CopyFcn=|
      | sdspfscope2([],[],[],'BlockCopy');
      | dspfixptcopycallback
      mask Help: web(dspbhelp);
      mask StyleString: checkbox,popup(Time|Frequency|User-defined),edit,checkbox,edit,edit,checkbox,edit,edit,checkbox,checkbox,checkbox,checkbox,checkbox,checkbox,checkbox,checkbox,edit,checkbox,popup(Hertz|rad/sec),popup([0...Fs/2]|[-Fs/2...Fs/2]|[0...Fs]),checkbox,edit,edit,popup(Magnitude|dB),edit,edit,edit,checkbox,edit,edit,edit,edit
      mask CallbackString: dspblkbfftscope2('dynamic','ScopeProperties')|||dspblkbfftscope2('dynamic','useBuffer');|||dspblkbfftscope2('dynamic','FftLenCheckbox');|||dspblkbfftscope2('dynamic','DisplayProperties');|||||||dspblkbfftscope2('dynamic','OpenScope');||dspblkbfftscope2('dynamic','AxisProperties');|||dspblkbfftscope2('dynamic','InheritXIncr');|||||||dspblkbfftscope2('dynamic','LineProperties');||||
      mask Display: plot(x,y); text(14,20,str);
  Zero-Order Hold : ZeroOrderHold  SampleTime=t_sample
  wires:
  Input/1 -> Zero-Order Hold/1
  Zero-Order Hold/1 -> Spectrum Scope/1(In1)

== system wt_blockset_beta/Mechanical Components/One-mass model  ==
  T_wt : Inport
  T_em : Inport  Port=2
  Gain1 : Gain  Gain=1/J  SaturateOnIntegerOverflow=on
  Gain2 : Gain  Gain=K  SaturateOnIntegerOverflow=on
  Gain3 : Gain  Gain=K  SaturateOnIntegerOverflow=on
  Gain4 : Gain  Gain=ModeOp  SaturateOnIntegerOverflow=on
  Integrator : Integrator  InitialCondition=init_speed  UpperSaturationLimit=0.95*2*pi*60  LowerSaturationLimit=0
  Sum : Sum  SaturateOnIntegerOverflow=on  InputSameDT=on
  omg_em : Outport  InitialOutput=0
  omg_wt : Outport  Port=2  InitialOutput=0
  wires:
  Gain1/1 -> Integrator/1
  Sum/1 -> Gain1/1
  T_em/1 -> Gain3/1
  T_wt/1 -> Gain4/1
  Integrator/1 -> omg_wt/1, Gain2/1
  Gain2/1 -> omg_em/1
  Gain3/1 -> Sum/2
  Gain4/1 -> Sum/1

== system wt_blockset_beta/Mechanical Components/Two-mass model ==
  T_wt : Inport
  T_em : Inport  Port=2
  Integrator : Integrator  InitialCondition=init(1)
  Integrator1 : Integrator
  Integrator2 : Integrator  InitialCondition=init(2)
  Integrator3 : Integrator
  Mux : Mux  Inputs=6
  domg_em/dt : Fcn  Expr=(-Dshaft*u(1)-Kshaft*u(2)+Dshaft*u(3)*Kgear+Kshaft*Kgear*u(4)+(Kgear^2)*u(6))/(Jem*Kgear^2)
  domg_wt/dt : Fcn  Expr=(Dshaft*u(1)/Kgear+Kshaft*u(2)/Kgear-Dshaft*u(3)-Kshaft*u(4)-u(5))/Jwt
  domg_wt/dt1 : Fcn  Expr=Dshaft*(u(1)/Kgear-u(3))+Kshaft*(u(2)/Kgear-u(4))
  omega_gen : Selector  Elements=[1]  InputPortWidth=6
  omega_gen1 : Selector  Elements=[1]  InputPortWidth=6
  omega_turbine : Selector  Elements=[3]  InputPortWidth=6
  omega_turbine1 : Selector  Elements=[3]  InputPortWidth=6
  omg_em : Outport
  T_shaft : Outport  Port=2
  omg_wt : Outport  Port=3
  wires:
  omega_turbine/1 -> omg_wt/1
  omega_gen/1 -> omg_em/1
  domg_wt/dt1/1 -> T_shaft/1
  T_em/1 -> Mux/6
  T_wt/1 -> Mux/5
  omega_turbine1/1 -> Integrator3/1
  domg_wt/dt/1 -> Integrator2/1
  omega_gen1/1 -> Integrator1/1
  domg_em/dt/1 -> Integrator/1
  Mux/1 -> omega_turbine/1, omega_gen/1, domg_wt/dt1/1, omega_turbine1/1, domg_wt/dt/1, omega_gen1/1, domg_em/dt/1
  Integrator3/1 -> Mux/4  "theta_wt"
  Integrator2/1 -> Mux/3  "omg_wt"
  Integrator1/1 -> Mux/2  "theta_em"
  Integrator/1 -> Mux/1  "omg_em"

== system wt_blockset_beta/Mechanical Components/Two-mass model 'C' S-Function ==
  T_wt : Inport
  T_em : Inport  Port=2
  Demux : Demux  Outputs=3
  Mux : Mux  Inputs=2
  S-Function : S-Function  FunctionName=torsional_torque  Parameters=Jem Jwt Kshaft Dshaft Kgear init_cond
  omg_em : Outport
  T_shaft : Outport  Port=2
  omg_wt : Outport  Port=3
  wires:
  Demux/3 -> T_shaft/1
  Demux/1 -> omg_em/1
  Demux/2 -> omg_wt/1
  S-Function/1 -> Demux/1
  T_em/1 -> Mux/2
  T_wt/1 -> Mux/1
  Mux/1 -> S-Function/1

== system wt_blockset_beta/Mechanical Components/Wind Model SB-1 ==
  omg_wt : Inport
  0 Harmonic Filter : TransferFcn  Numerator=[0 4.7869*d 0.9904]  Denominator=[7.6823*d^2 7.3518*d 1]
  3 Harmonic : Sum  SaturateOnIntegerOverflow=on  InputSameDT=on
  3 Harmonic Filter_1 : TransferFcn  Numerator=[0 0.2766*d 0.0307]  Denominator=[0.3691*d^2 1.7722*d 1]
  3 Harmonic Filter_2 : TransferFcn  Numerator=[0 0.2766*d 0.0307]  Denominator=[0.3691*d^2 1.7722*d 1]
  Clock : Clock
  Constant1 : Constant  Value=v_mean
  Kaimal_Filter_1 : Subsystem
  Kaimal_Filter_2 : Subsystem
  Kaimal_Filter_3 : Subsystem
  Mux : Mux  Inputs=2
  Product : Product  SaturateOnIntegerOverflow=on  InputSameDT=on
  Product1 : Product  SaturateOnIntegerOverflow=on  InputSameDT=on
  Sum : Sum  SaturateOnIntegerOverflow=on  InputSameDT=on
  Sum2 : Sum  SaturateOnIntegerOverflow=on  InputSameDT=on
  Unit Delay : UnitDelay  SampleTime=T_sample
  Unit Delay1 : UnitDelay  SampleTime=T_sample
  White Noise_1 : Subsystem  mask(Continuous White Noise.){Cov=[1], Ts=T_sample, seed=[256]}
      mask prompts: Cov "Noise Power:"; Ts "Sample Time:"
      mask help:
      | White noise for continuous (s-domain) systems.
      | Band-limited using zero-order-hold.
      mask init:
      | r = rand(1,12); r2 = [r(1),r;r,r(12)]; t =[1:13;1:13];
      mask Help: Implemented using white noise into Zero-Order Hold block. The seed and power can be vectors of the same length to produce a vector of white noise sources. For faster simulation, set sample time to the highest value possible but in accordance with the fastest dynamics of system.
      mask Display: plot(t(:),r2(:))
  White Noise_2 : Subsystem  mask(Continuous White Noise.){@1=[1], @2=T_sample, @3=[894]}
      mask prompts: @1 "Noise Power:"; @2 "Sample Time:"; @3 "Seed"
      mask help:
      | White noise for continuous (s-domain) systems.
      | Band-limited using zero-order-hold.
      mask init:
      | Cov = @1; Ts = @2; seed = @3; r = rand(1,12); r2 = [r(1),r;r,r(12)]; t =[1:13;1:13];
      mask Help: Implemented using white noise into Zero-Order Hold block. The seed and power can be vectors of the same length to produce a vector of white noise sources. For faster simulation, set sample time to the highest value possible but in accordance with the fastest dynamics of system.
      mask Display: plot(t(:),r2(:))
  White Noise_3 : Subsystem  mask(Continuous White Noise.){@1=[1], @2=T_sample, @3=[31]}
      mask prompts: @1 "Noise Power:"; @2 "Sample Time:"; @3 "Seed"
      mask help:
      | White noise for continuous (s-domain) systems.
      | Band-limited using zero-order-hold.
      mask init:
      | Cov = @1; Ts = @2; seed = @3; r = rand(1,12); r2 = [r(1),r;r,r(12)]; t =[1:13;1:13];
      mask Help: Implemented using white noise into Zero-Order Hold block. The seed and power can be vectors of the same length to produce a vector of white noise sources. For faster simulation, set sample time to the highest value possible but in accordance with the fastest dynamics of system.
      mask Display: plot(t(:),r2(:))
  cos fun : Fcn  Expr=sqrt(2)*cos(3*u[1]*u[2])
  sin fun : Fcn  Expr=sqrt(2)*sin(3*u[1]*u[2])
  wind : Outport  InitialOutput=[u0]
  wires:
  Kaimal_Filter_2/1(out_1) -> 3 Harmonic Filter_1/1
  Kaimal_Filter_3/1(out_1) -> 3 Harmonic Filter_2/1
  cos fun/1 -> Unit Delay/1
  sin fun/1 -> Unit Delay1/1
  Product/1 -> 3 Harmonic/1
  Product1/1 -> 3 Harmonic/2
  3 Harmonic Filter_2/1 -> Product1/2
  3 Harmonic/1 -> Sum/2
  0 Harmonic Filter/1 -> Sum2/2
  Sum2/1 -> Sum/1
  Constant1/1 -> Sum2/1
  Sum/1 -> wind/1
  Kaimal_Filter_1/1(out_1) -> 0 Harmonic Filter/1
  White Noise_1/1(Out_1) -> Kaimal_Filter_1/1(in_1)
  White Noise_2/1(Out_1) -> Kaimal_Filter_2/1(in_1)
  White Noise_3/1(Out_1) -> Kaimal_Filter_3/1(in_1)
  3 Harmonic Filter_1/1 -> Product/1
  Mux/1 -> cos fun/1, sin fun/1
  omg_wt/1 -> Mux/1
  Unit Delay/1 -> Product/2
  Unit Delay1/1 -> Product1/1
  Clock/1 -> Mux/2
